simulink model "math_sqrt_test_tmp"  (Simulink 8.3)
settings: Solver=VariableStepDiscrete  StartTime=0.0  StopTime=10.0  RelTol=1e-3
undefined symbols (not defined in the file): Newton, Raphson
libraries: simulink x2
settings Model: Creator=arnaud  LastModifiedBy=hbourbou
settings DataIOCC: SaveFormat=Structure
settings OptimizationCC: ExpressionDepthLimit=2147483647
settings DebuggingCC: FcnCallInpInsideContextMsg=EnableAllAsWarning  FrameProcessingCompatibilityMsg=error

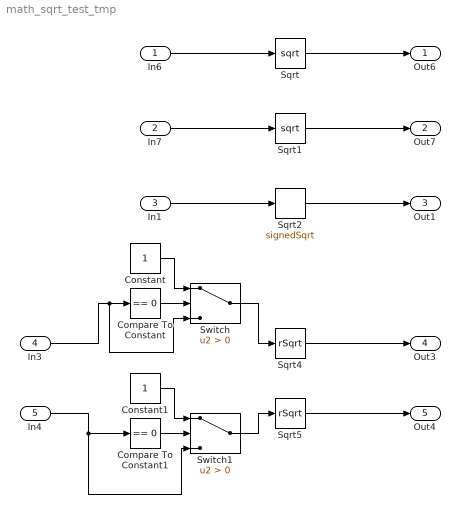
== system math_sqrt_test_tmp ==
  In6 : Inport  OutDataTypeStr=uint32
  In7 : Inport  Port=2  OutDataTypeStr=uint32
  In1 : Inport  Port=3
  In3 : Inport  Port=4  OutDataTypeStr=double
  In4 : Inport  Port=5  OutDataTypeStr=uint32
  Compare To Constant : simulink/Logic and Bit Operations/Compare To Constant  relop===  const=0  OutDataTypeStr=boolean
  Compare To Constant1 : simulink/Logic and Bit Operations/Compare To Constant  relop===  const=0  OutDataTypeStr=boolean
  Constant : Constant
  Constant1 : Constant
  Sqrt : Sqrt  SaturateOnIntegerOverflow=on
  Sqrt1 : Sqrt  SaturateOnIntegerOverflow=on
  Sqrt2 : Sqrt  Operator=signedSqrt  SaturateOnIntegerOverflow=on
  Sqrt4 : Sqrt  Operator=rSqrt  SaturateOnIntegerOverflow=on
  Sqrt5 : Sqrt  Operator=rSqrt  AlgorithmType=Newton-Raphson  SaturateOnIntegerOverflow=on
  Switch : Switch  Criteria=u2 > Threshold
  Switch1 : Switch  Criteria=u2 > Threshold
  Out6 : Outport
  Out7 : Outport  Port=2
  Out1 : Outport  Port=3
  Out3 : Outport  Port=4
  Out4 : Outport  Port=5
  wires:
  In6/1 -> Sqrt/1
  Sqrt/1 -> Out6/1
  In7/1 -> Sqrt1/1
  Sqrt1/1 -> Out7/1
  In1/1 -> Sqrt2/1
  Sqrt2/1 -> Out1/1
  Sqrt4/1 -> Out3/1
  Sqrt5/1 -> Out4/1
  In3/1 -> Switch/3, Compare To Constant/1
  Compare To Constant/1 -> Switch/2
  Constant/1 -> Switch/1
  Switch/1 -> Sqrt4/1
  In4/1 -> Compare To Constant1/1, Switch1/3
  Compare To Constant1/1 -> Switch1/2
  Constant1/1 -> Switch1/1
  Switch1/1 -> Sqrt5/1
